simulink model "Aufgabe2_2"  (Simulink 10.0)
settings: Solver=VariableStepAuto  StartTime=0.0  StopTime=10.0  RelTol=1e-3
values from neighbouring files (symbols this model uses):
  H = inv(A)*(Phi - eye(3)) * B    [Auf_2_2_Initialisierung.m]
  Phi = expm(A*Ta)    [Auf_2_2_Initialisierung.m]
undefined symbols (not defined in the file or in its folder): C, D
libraries: cstblocks x1
settings Model: Creator=kirch  LastModifiedBy=kirch
settings DataIOCC: SaveFormat=Dataset  ReturnWorkspaceOutputs=on
settings OptimizationCC: LifeSpan=auto
settings DebuggingCC: UnderspecifiedInitializationDetection=Simplified  MergeDetectMultiDrivingBlocksExec=error  SFUnexpectedBacktrackingDiag=error  SFNoUnconditionalDefaultTransitionDiag=error  SFExecutionAtInitializationDiag=warning  ArithmeticOperatorsInVariantConditions=error
settings HardwareCC: ProdBitPerPointer=64  ProdBitPerSizeT=64  ProdBitPerPtrDiffT=64  ProdLargestAtomicFloat=Float  ProdIntDivRoundTo=Zero  ProdEndianess=LittleEndian  ProdWordSize=64  ProdHWDeviceType=Intel->x86-64 (Windows64)
settings ModelReferenceCC: PropagateSignalLabelsOutOfModel=on
settings SFSimCC: SimUseLocalCustomCode=on  CustomCodeUndefinedFunction=FilterOut
settings RTWCC: RTWUseLocalCustomCode=on
settings CodeAppCC: StateflowObjectComments=off
settings GRTTargetCC: TargetLangStandard=C99 (ISO)  CombineOutputUpdateFcns=on  GRTInterface=off
settings ConfigComp: CovMetricSettings=dwe  CovHtmlReporting=off  CovSaveCumulativeToWorkspaceVar=off  CovSaveSingleToWorkspaceVar=off

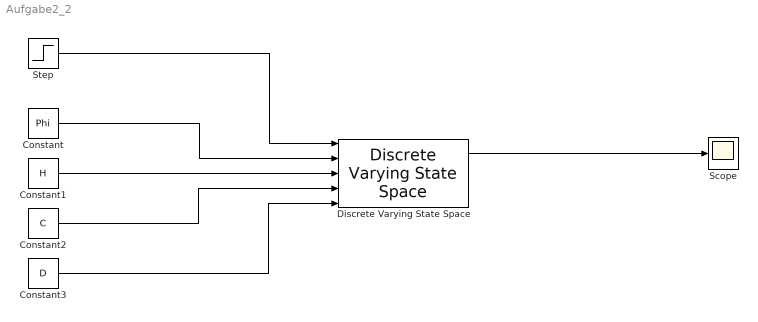
== system Aufgabe2_2 ==
  Constant : Constant  Value=Phi  VectorParams1D=off
  Constant1 : Constant  Value=H  VectorParams1D=off
  Constant2 : Constant  Value=C  VectorParams1D=off
  Constant3 : Constant  Value=D  VectorParams1D=off
  Discrete Varying State Space : cstblocks/Linear Parameter Varying/Discrete Varying State Space  x0=0  Ts=15e-3  OutputX=on  OutputDX=on
      settings: SourceProductName=Control System Toolbox  SourceProductBaseCode=CT
  Scope : Scope
  Step : Step  After=0.2  SampleTime=0
  wires:
  Constant/1 -> Discrete Varying State Space/2
  Constant1/1 -> Discrete Varying State Space/3
  Constant2/1 -> Discrete Varying State Space/4
  Constant3/1 -> Discrete Varying State Space/5
  Step/1 -> Discrete Varying State Space/1
  Discrete Varying State Space/1 -> Scope/1
